simulink model "altitudecontroller"  (R2017a)
settings: Solver=VariableStepAuto  StartTime=0.0  StopTime=10  RelTol=1e-3
libraries: simulink x6
settings Model: Creator=jdeka  LastModifiedBy=jdeka

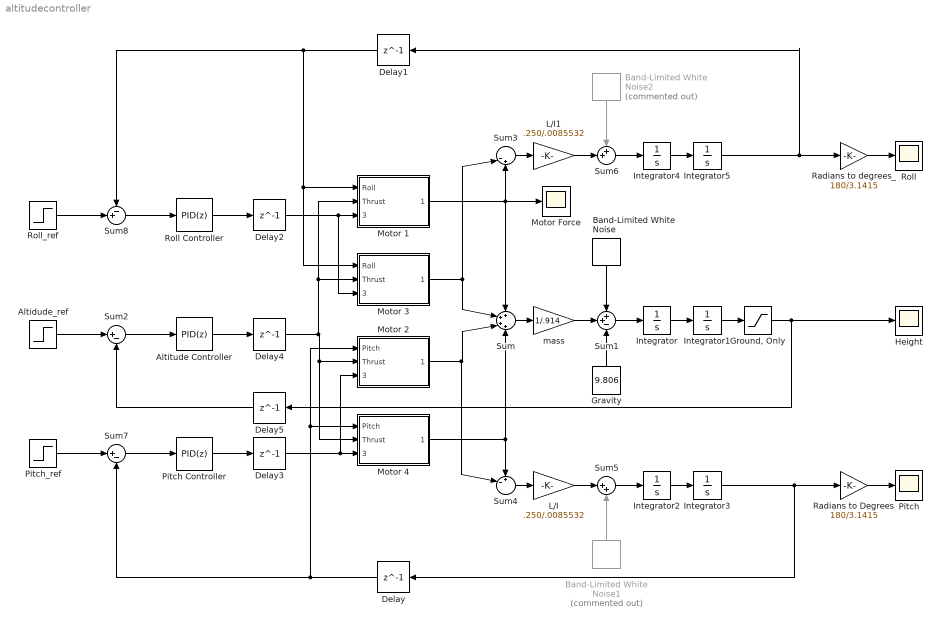
== system altitudecontroller ==
  Altidude_ref : Step  Time=0  SampleTime=0
  Altitude Controller : simulink/Continuous/PID Controller  Controller=PID  TimeDomain=Discrete-time  SampleTime=.01  IntegratorMethod=Forward Euler  FilterMethod=Forward Euler  Form=Parallel  UseFilter=off  ControllerParametersSource=internal  P=100  I=12  D=55  N=100  InitialConditionSource=internal  InitialConditionForIntegrator=0  InitialConditionForFilter=0  ExternalReset=none  LimitOutput=off  UpperSaturationLimit=inf  LowerSaturationLimit=-inf  LinearizeAsGain=off  AntiWindupMode=none  Kb=1  TrackingMode=off  Kt=1  PParamMin=[]  PParamMax=[]  IParamMin=[]  IParamMax=[]  DParamMin=[]  DParamMax=[]  NParamMin=[]  NParamMax=[]  KbParamMin=[]  KbParamMax=[]  KtParamMin=[]  KtParamMax=[]  POutMin=[]  POutMax=[]  IOutMin=[]  IOutMax=[]  DOutMin=[]  DOutMax=[]  NOutMin=[]  NOutMax=[]  KbOutMin=[]  KbOutMax=[]  KtOutMin=[]  KtOutMax=[]  IntegratorOutMin=[]  IntegratorOutMax=[]  FilterOutMin=[]  FilterOutMax=[]  SumOutMin=[]  SumOutMax=[]  SumI1OutMin=[]  SumI1OutMax=[]  SumI2OutMin=[]  SumI2OutMax=[]  SumI3OutMin=[]  SumI3OutMax=[]  SumDOutMin=[]  SumDOutMax=[]  SaturationOutMin=[]  SaturationOutMax=[]  IntegratorContinuousStateAttributes=''  IntegratorStateMustResolveToSignalObject=off  IntegratorRTWStateStorageClass=Auto  FilterContinuousStateAttributes=''  FilterStateMustResolveToSignalObject=off  FilterRTWStateStorageClass=Auto  DifferentiatorICPrevScaledInput=0  DifferentiatorOutMin=[]  DifferentiatorOutMax=[]  InitialConditionSetting=State (most efficient)
  Band-Limited White Noise : simulink/Sources/Band-Limited White Noise  Cov=.1  Ts=.01  seed=[24541]
  Band-Limited White Noise1 : simulink/Sources/Band-Limited White Noise  Commented=on  Cov=[0.1]  Ts=0.1  seed=[23341]
  Band-Limited White Noise2 : simulink/Sources/Band-Limited White Noise  Commented=on  Cov=.2  Ts=.01  seed=[23111]
  Delay{,1..5} (6 alike) : Delay  DelayLength=1
  Gravity : Constant  Value=9.806
  "Ground, Only " : Saturate  UpperLimit=inf  LowerLimit=0
  Height : Scope
  Integrator{,1..5} (6 alike) : Integrator
  L/I : Gain  Gain=.250/.0085532
  L/I1 : Gain  Gain=.250/.0085532
  Motor 1 : Subsystem
  Motor 2 : Subsystem
  Motor 3 : Subsystem
  Motor 4 : Subsystem
  Motor Force : Scope
  Pitch : Scope
  Pitch Controller : simulink/Continuous/PID Controller  Controller=PID  TimeDomain=Discrete-time  SampleTime=.01  IntegratorMethod=Forward Euler  FilterMethod=Forward Euler  Form=Parallel  UseFilter=off  ControllerParametersSource=internal  P=0  I=0  D=0  N=100  InitialConditionSource=internal  InitialConditionForIntegrator=0  InitialConditionForFilter=0  ExternalReset=none  LimitOutput=off  UpperSaturationLimit=inf  LowerSaturationLimit=-inf  LinearizeAsGain=off  AntiWindupMode=none  Kb=1  TrackingMode=off  Kt=1  PParamMin=[]  PParamMax=[]  IParamMin=[]  IParamMax=[]  DParamMin=[]  DParamMax=[]  NParamMin=[]  NParamMax=[]  KbParamMin=[]  KbParamMax=[]  KtParamMin=[]  KtParamMax=[]  POutMin=[]  POutMax=[]  IOutMin=[]  IOutMax=[]  DOutMin=[]  DOutMax=[]  NOutMin=[]  NOutMax=[]  KbOutMin=[]  KbOutMax=[]  KtOutMin=[]  KtOutMax=[]  IntegratorOutMin=[]  IntegratorOutMax=[]  FilterOutMin=[]  FilterOutMax=[]  SumOutMin=[]  SumOutMax=[]  SumI1OutMin=[]  SumI1OutMax=[]  SumI2OutMin=[]  SumI2OutMax=[]  SumI3OutMin=[]  SumI3OutMax=[]  SumDOutMin=[]  SumDOutMax=[]  SaturationOutMin=[]  SaturationOutMax=[]  IntegratorContinuousStateAttributes=''  IntegratorStateMustResolveToSignalObject=off  IntegratorRTWStateStorageClass=Auto  FilterContinuousStateAttributes=''  FilterStateMustResolveToSignalObject=off  FilterRTWStateStorageClass=Auto  DifferentiatorICPrevScaledInput=0  DifferentiatorOutMin=[]  DifferentiatorOutMax=[]  InitialConditionSetting=State (most efficient)
  Pitch_ref : Step  Time=0  After=0  SampleTime=0
  Radians to Degrees : Gain  Gain=180/3.1415
  Radians to degrees_ : Gain  Gain=180/3.1415
  Roll : Scope
  Roll Controller : simulink/Continuous/PID Controller  Controller=PID  TimeDomain=Discrete-time  SampleTime=.01  IntegratorMethod=Forward Euler  FilterMethod=Forward Euler  Form=Parallel  UseFilter=off  ControllerParametersSource=internal  P=0  I=0  D=0  N=100  InitialConditionSource=internal  InitialConditionForIntegrator=0  InitialConditionForFilter=0  ExternalReset=none  LimitOutput=off  UpperSaturationLimit=inf  LowerSaturationLimit=-inf  LinearizeAsGain=off  AntiWindupMode=none  Kb=1  TrackingMode=off  Kt=1  PParamMin=[]  PParamMax=[]  IParamMin=[]  IParamMax=[]  DParamMin=[]  DParamMax=[]  NParamMin=[]  NParamMax=[]  KbParamMin=[]  KbParamMax=[]  KtParamMin=[]  KtParamMax=[]  POutMin=[]  POutMax=[]  IOutMin=[]  IOutMax=[]  DOutMin=[]  DOutMax=[]  NOutMin=[]  NOutMax=[]  KbOutMin=[]  KbOutMax=[]  KtOutMin=[]  KtOutMax=[]  IntegratorOutMin=[]  IntegratorOutMax=[]  FilterOutMin=[]  FilterOutMax=[]  SumOutMin=[]  SumOutMax=[]  SumI1OutMin=[]  SumI1OutMax=[]  SumI2OutMin=[]  SumI2OutMax=[]  SumI3OutMin=[]  SumI3OutMax=[]  SumDOutMin=[]  SumDOutMax=[]  SaturationOutMin=[]  SaturationOutMax=[]  IntegratorContinuousStateAttributes=''  IntegratorStateMustResolveToSignalObject=off  IntegratorRTWStateStorageClass=Auto  FilterContinuousStateAttributes=''  FilterStateMustResolveToSignalObject=off  FilterRTWStateStorageClass=Auto  DifferentiatorICPrevScaledInput=0  DifferentiatorOutMin=[]  DifferentiatorOutMax=[]  InitialConditionSetting=State (most efficient)
  Roll_ref : Step  Time=0  After=2*3.1415/180  SampleTime=0
  Sum : Sum  Inputs=++++
  Sum1 : Sum  Inputs=++-
  Sum2 : Sum  Inputs=|+-
  Sum3 : Sum  Inputs=||-+
  Sum4 : Sum  Inputs=+-||
  Sum5 : Sum  Inputs=|++
  Sum6 : Sum  Inputs=++|
  Sum7 : Sum  Inputs=|+-
  Sum8 : Sum  Inputs=-+|
  mass : Gain  Gain=1/.914
  wires:
  Integrator/1 -> Integrator1/1
  Sum/1 -> mass/1
  Sum1/1 -> Integrator/1
  Integrator1/1 -> "Ground, Only "/1
  Motor 1/1(Motor out) -> Motor Force/1, Sum/1, Sum3/2
  Motor 3/1(Motor out) -> Sum3/1, Sum/2
  Motor 2/1(Motor out) -> Sum4/2, Sum/3
  Motor 4/1(Motor out) -> Sum/4, Sum4/1
  Band-Limited White Noise/1 -> Sum1/1
  Gravity/1 -> Sum1/3
  mass/1 -> Sum1/2
  Sum5/1 -> Integrator2/1
  Integrator2/1 -> Integrator3/1
  L/I/1 -> Sum5/1
  Band-Limited White Noise1/1 -> Sum5/2
  Sum4/1 -> L/I/1
  Sum6/1 -> Integrator4/1
  Band-Limited White Noise2/1 -> Sum6/1
  Integrator4/1 -> Integrator5/1
  Sum3/1 -> L/I1/1
  L/I1/1 -> Sum6/2
  Roll Controller/1 -> Delay2/1
  Pitch Controller/1 -> Delay3/1
  Altitude Controller/1 -> Delay4/1
  Sum7/1 -> Pitch Controller/1
  Sum2/1 -> Altitude Controller/1
  Sum8/1 -> Roll Controller/1
  Roll_ref/1 -> Sum8/2
  Pitch_ref/1 -> Sum7/1
  Altidude_ref/1 -> Sum2/1
  "Ground, Only "/1 -> Delay5/1, Height/1
  Integrator3/1 -> Radians to Degrees/1, Delay/1
  Integrator5/1 -> Radians to degrees_/1, Delay1/1
  Radians to Degrees/1 -> Pitch/1
  Radians to degrees_/1 -> Roll/1
  Delay/1 -> Sum7/2, Motor 2/1(Pitch), Motor 4/1(Pitch)
  Delay1/1 -> Sum8/1, Motor 3/1(Roll), Motor 1/1(Roll)
  Delay2/1 -> Motor 3/3(Roll Control), Motor 1/3(Roll Control)
  Delay3/1 -> Motor 2/3(Pitch Control), Motor 4/3(Pitch Control)
  Delay4/1 -> Motor 2/2(Thrust), Motor 4/2(Thrust), Motor 1/2(Thrust), Motor 3/2(Thrust)
  Delay5/1 -> Sum2/2

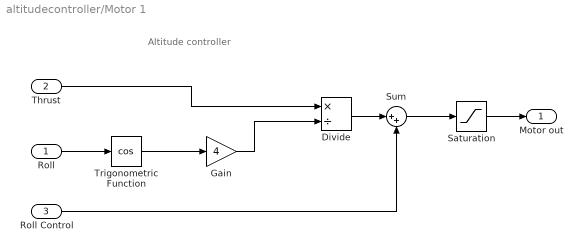
== system altitudecontroller/Motor 1 ==
  note: Altitude controller
  Roll : Inport
  Thrust : Inport  Port=2
  Roll Control : Inport  Port=3
  Divide : Product  Inputs=*/
  Gain : Gain  Gain=4
  Saturation : Saturate  UpperLimit=5.814  LowerLimit=0.1
  Sum : Sum  Inputs=|++
  Trigonometric Function : Trigonometry  Operator=cos
  Motor out : Outport
  wires:
  Gain/1 -> Divide/2
  Roll/1 -> Trigonometric Function/1
  Trigonometric Function/1 -> Gain/1
  Thrust/1 -> Divide/1
  Divide/1 -> Sum/1
  Saturation/1 -> Motor out/1
  Sum/1 -> Saturation/1
  Roll Control/1 -> Sum/2

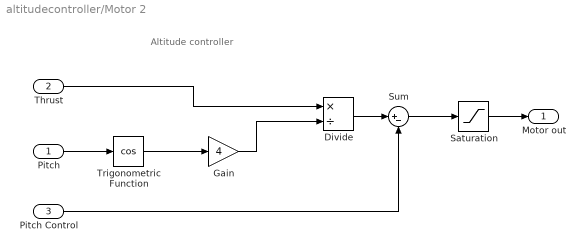
== system altitudecontroller/Motor 2 ==
  note: Altitude controller
  Pitch : Inport
  Thrust : Inport  Port=2
  Pitch Control : Inport  Port=3
  Divide : Product  Inputs=*/
  Gain : Gain  Gain=4
  Saturation : Saturate  UpperLimit=5.814  LowerLimit=0.1
  Sum : Sum  Inputs=|+-
  Trigonometric Function : Trigonometry  Operator=cos
  Motor out : Outport
  wires:
  Gain/1 -> Divide/2
  Pitch/1 -> Trigonometric Function/1
  Trigonometric Function/1 -> Gain/1
  Thrust/1 -> Divide/1
  Divide/1 -> Sum/1
  Saturation/1 -> Motor out/1
  Sum/1 -> Saturation/1
  Pitch Control/1 -> Sum/2

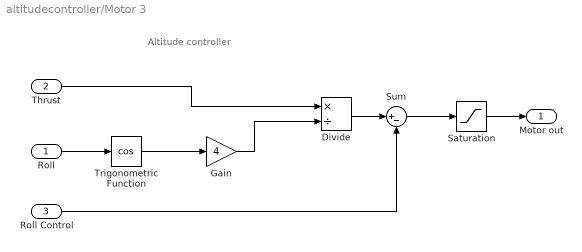
== system altitudecontroller/Motor 3 ==
  note: Altitude controller
  Roll : Inport
  Thrust : Inport  Port=2
  Roll Control : Inport  Port=3
  Divide : Product  Inputs=*/
  Gain : Gain  Gain=4
  Saturation : Saturate  UpperLimit=5.814  LowerLimit=0.1
  Sum : Sum  Inputs=|+-
  Trigonometric Function : Trigonometry  Operator=cos
  Motor out : Outport
  wires:
  Gain/1 -> Divide/2
  Roll/1 -> Trigonometric Function/1
  Trigonometric Function/1 -> Gain/1
  Thrust/1 -> Divide/1
  Divide/1 -> Sum/1
  Saturation/1 -> Motor out/1
  Sum/1 -> Saturation/1
  Roll Control/1 -> Sum/2

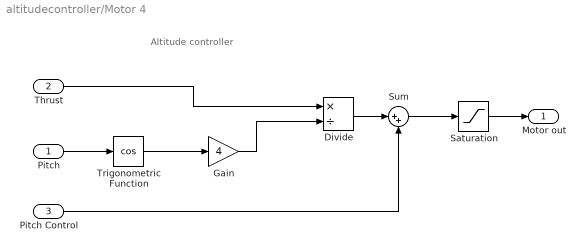
== system altitudecontroller/Motor 4 ==
  note: Altitude controller
  Pitch : Inport
  Thrust : Inport  Port=2
  Pitch Control : Inport  Port=3
  Divide : Product  Inputs=*/
  Gain : Gain  Gain=4
  Saturation : Saturate  UpperLimit=5.814  LowerLimit=0.1
  Sum : Sum  Inputs=|++
  Trigonometric Function : Trigonometry  Operator=cos
  Motor out : Outport
  wires:
  Gain/1 -> Divide/2
  Pitch/1 -> Trigonometric Function/1
  Trigonometric Function/1 -> Gain/1
  Thrust/1 -> Divide/1
  Divide/1 -> Sum/1
  Saturation/1 -> Motor out/1
  Sum/1 -> Saturation/1
  Pitch Control/1 -> Sum/2
